simulink model "Xcvr_SSB_AM_2p5"  (Simulink 8.0)
settings: Solver=VariableStepDiscrete  SolverMode=SingleTasking  StartTime=0.0  StopTime=10  RelTol=1e-3
PreLoadFcn:
  | Fs=80e6;
  | 
  | phee=da_rom();
  | [phee_1,phee_2]=da_i2_rom();
  | 
  | Dcic=64;       % CIC decimation
  | Dfac=128;    % following DA filter decimation
  | N = 6;           %       (2^(N+1))=Dfac
  | Daudio=Dcic*Dfac;
  | Faudio=Fs/Daudio;
  | 
  | load info_filt_ssb_4
  | load Serial_Intfc_Stream_5
  | 
  | % AGC related
  | x=0.5:1/256:(1-1/256);
  | addr=(x-0.5)*256;
  | y=1./x;
values from neighbouring files (symbols this model uses):
  Serial_Interface = [0 0 0 0 0 0 0 0 0 0 0 0 ... (11390 elements, 2x5695)]    [Serial_Intfc_Stream_5.mat]
undefined symbols (not defined in the file or in its folder): get, sided, Two, xlipgetpartsetting
undefined symbols (not defined in the file): ssb_coef
libraries: xbsIndex_r4 x1307, dspsrcs4 x5, simulink x2, dspsigops x2, dspsnks4 x1
(part 1 of 11)
settings Model: Creator=dbenson  LastModifiedBy=user
settings DataIOCC: SignalLoggingSaveFormat=ModelDataLogs
settings OptimizationCC: InitFltsAndDblsToZero=on
settings DebuggingCC: FcnCallInpInsideContextMsg=UseLocalSettings  StrictBusMsg=ErrorOnBusTreatedAsVector
settings GRTTargetCC: CombineOutputUpdateFcns=off  GRTInterface=on

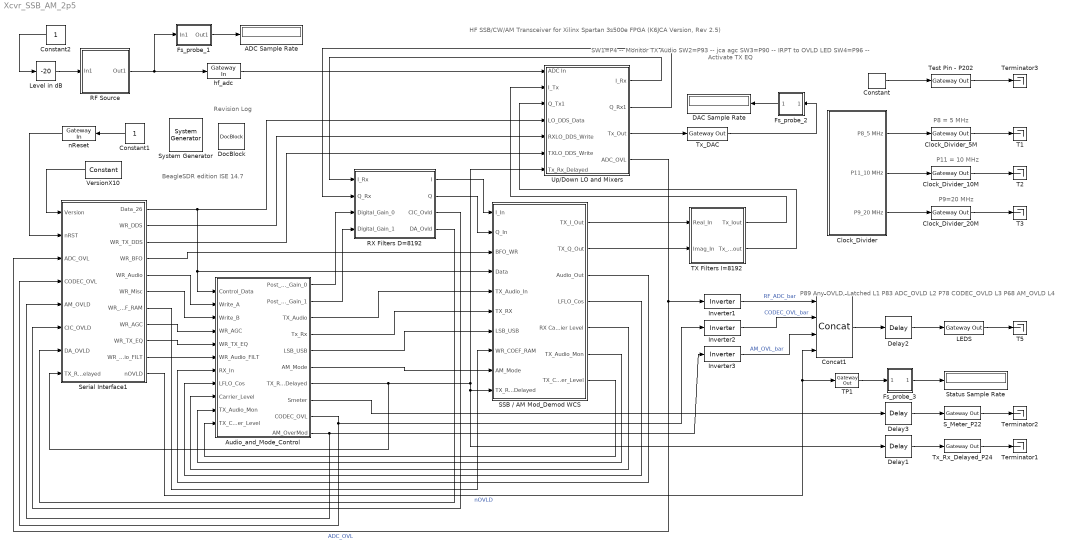
== system Xcvr_SSB_AM_2p5 ==
  note: HF SSB/CW/AM Transceiver for Xilinx Spartan 3s500e FPGA
      | (K6JCA Version, Rev 2.5)
  note: BeagleSDR edition ISE 14.7
  note: SW1=P4 -- Monitor TX Audio
      | SW2=P93 -- jca agc
      | SW3=P90 -- IRPT to OVLD LED
      | SW4=P96 -- Activate TX EQ
  note: P8 = 5 MHz
  note: P11 = 10 MHz
  note: P9=20 MHz
  note: P89  Any OVLD, Latched L1
      | P83  ADC_OVLD L2
      | P78  CODEC_OVLD L3
      | P68  AM_OVLD  L4
  note: Revision
      | Log
  " System Generator" : xbsIndex_r4/ System Generator  Tag=genX  xilinxfamily=spartan3e  part=xc3s500e  speed=-4  package=pq208  synthesis_tool=XST  clock_wrapper=Expose Clock Ports  directory=./netlist_2p5  proj_type=Project Navigator  Synth_file=XST Defaults  Impl_file=ISE Defaults  testbench=off  simulink_period=1/(32*Fs)  sysclk_period=20  dcm_input_clock_period=100  incr_netlist=off  trim_vbits=Everywhere in SubSystem  dbl_ovrd=According to Block Masks  core_generation=According to Block Masks  run_coregen=off  deprecated_control=off  eval_field=0  block_type=sysgen
      settings: block_version=9.2.00
  ADC Sample Rate : Display
  Audio_and_Mode_Control : Subsystem
  Clock_Divider : Subsystem
  Clock_Divider_10M : xbsIndex_r4/Gateway Out  inherit_from_input=off  hdl_port=on  timing_constraint=None  locs_specified=on  LOCs={'P11'}  UseAsDAC=off  DACChannel='1'  block_type=gatewayout
      settings: infoedit="Gateway out block.  Converts Xilinx fixed point inputs into ouputs of type Simulink integer, double, or fixed point.<br><br>Hardware notes:  In hardware these blocks become top level output ports or are discarded, depending on how they are configured."  block_version=12.1
  Clock_Divider_20M : xbsIndex_r4/Gateway Out  inherit_from_input=off  hdl_port=on  timing_constraint=None  locs_specified=on  LOCs={'P9'}  UseAsDAC=off  DACChannel='1'  block_type=gatewayout
      settings: infoedit="Gateway out block.  Converts Xilinx fixed point inputs into ouputs of type Simulink integer, double, or fixed point.<br><br>Hardware notes:  In hardware these blocks become top level output ports or are discarded, depending on how they are configured."  block_version=12.1
  Clock_Divider_5M : xbsIndex_r4/Gateway Out  inherit_from_input=off  hdl_port=on  timing_constraint=None  locs_specified=on  LOCs={'P8'}  UseAsDAC=off  DACChannel='1'  block_type=gatewayout
      settings: infoedit="Gateway out block.  Converts Xilinx fixed point inputs into ouputs of type Simulink integer, double, or fixed point.<br><br>Hardware notes:  In hardware these blocks become top level output ports or are discarded, depending on how they are configured."  block_version=12.1
  Concat1 : xbsIndex_r4/Concat  num_inputs=4  dbl_ovrd=off  block_type=concat
      settings: block_version=12.1
  Constant : xbsIndex_r4/Constant  const=0  gui_display_data_type=Fixed-point  arith_type=Boolean  n_bits=1  bin_pt=0  preci_type=Single  exp_width=8  frac_width=24  explicit_period=off  period=1  equ=P=C  opselect=C  inp2=PCIN>>17  opr=+  inp1=P  carry=CIN  dbl_ovrd=off  block_type=constant
      settings: block_version=12.1
  Constant1 : Constant
  Constant2 : Constant
  DAC Sample Rate : Display
  Delay1 : xbsIndex_r4/Delay  rst=off  infoeditControl=Selection of Reset will increase slice count due to use of real FFs and instead of SRLs  en=off  latency=1  dbl_ovrd=off  reg_retiming=off  block_type=delay
      settings: block_version=12.1
  Delay2 : xbsIndex_r4/Delay  rst=off  infoeditControl=Selection of Reset will increase slice count due to use of real FFs and instead of SRLs  en=off  latency=1  dbl_ovrd=off  reg_retiming=off  block_type=delay
      settings: block_version=12.1
  Delay3 : xbsIndex_r4/Delay  rst=off  infoeditControl=Selection of Reset will increase slice count due to use of real FFs and instead of SRLs  en=off  latency=1  dbl_ovrd=off  reg_retiming=off  block_type=delay
      settings: block_version=12.1
  DocBlock : simulink/Model-Wide Utilities/DocBlock  DocumentType=Text
  Fs_probe_1 : Subsystem
  Fs_probe_2 : Subsystem
  Fs_probe_3 : Subsystem
  Inverter1 : xbsIndex_r4/Inverter  en=off  latency=0  dbl_ovrd=off  block_type=inv
      settings: block_version=12.1
  Inverter2 : xbsIndex_r4/Inverter  en=off  latency=0  dbl_ovrd=off  block_type=inv
      settings: block_version=12.1
  Inverter3 : xbsIndex_r4/Inverter  en=off  latency=0  dbl_ovrd=off  block_type=inv
      settings: block_version=12.1
  LEDS : xbsIndex_r4/Gateway Out  inherit_from_input=off  hdl_port=on  timing_constraint=None  locs_specified=on  LOCs={'P89','P83','P78','P68'}  UseAsDAC=off  DACChannel='1'  block_type=gatewayout
      settings: infoedit="Gateway out block.  Converts Xilinx fixed point inputs into ouputs of type Simulink integer, double, or fixed point.<br><br>Hardware notes:  In hardware these blocks become top level output ports or are discarded, depending on how they are configured."  block_version=12.1
  Level in dB : simulink/Math Operations/Slider Gain  low=-100  gain=-20  high=0
  RF Source : Subsystem
  RX Filters D=8192 : Subsystem
  SSB / AM Mod_Demod WCS : Subsystem
  S_Meter_P22 : xbsIndex_r4/Gateway Out  inherit_from_input=off  hdl_port=on  timing_constraint=None  locs_specified=on  LOCs={'P22'}  UseAsDAC=off  DACChannel='1'  block_type=gatewayout
      settings: infoedit="Gateway out block.  Converts Xilinx fixed point inputs into ouputs of type Simulink integer, double, or fixed point.<br><br>Hardware notes:  In hardware these blocks become top level output ports or are discarded, depending on how they are configured."  block_version=9.2.00
  Serial Interface1 : Subsystem
  Status Sample Rate : Display
  T{1..3,5} (4 alike) : Terminator
  TP1 : xbsIndex_r4/Gateway Out  inherit_from_input=off  hdl_port=off  timing_constraint=None  locs_specified=off  LOCs={ 'b15','c15','c16','d14','b4','e13','k1','g1'}  UseAsDAC=off  DACChannel='1'  block_type=gatewayout
      settings: infoedit="Gateway out block.  Converts Xilinx fixed point inputs into ouputs of type Simulink integer, double, or fixed point.<br><br>Hardware notes:  In hardware these blocks become top level output ports or are discarded, depending on how they are configured."  block_version=9.2.00
  TX Filters I=8192 : Subsystem
  Terminator1 : Terminator
  Terminator2 : Terminator
  Terminator3 : Terminator
  Test Pin - P202 : xbsIndex_r4/Gateway Out  inherit_from_input=off  hdl_port=on  timing_constraint=None  locs_specified=on  LOCs={ 'P202'}  UseAsDAC=off  DACChannel='1'  block_type=gatewayout
      settings: infoedit="Gateway out block.  Converts Xilinx fixed point inputs into ouputs of type Simulink integer, double, or fixed point.<br><br>Hardware notes:  In hardware these blocks become top level output ports or are discarded, depending on how they are configured."  block_version=9.2.00
  Tx_DAC : xbsIndex_r4/Gateway Out  inherit_from_input=off  hdl_port=on  timing_constraint=None  locs_specified=on  LOCs={'P55','P50','P61','P60','P63','P62','P65','P64','P74','P69','P76','P75','P82','P77'}  UseAsDAC=off  DACChannel='1'  block_type=gatewayout
      settings: infoedit="Gateway out block.  Converts Xilinx fixed point inputs into ouputs of type Simulink integer, double, or fixed point.<br><br>Hardware notes:  In hardware these blocks become top level output ports or are discarded, depending on how they are configured."  block_version=12.1
  Tx_Rx_Delayed_P24 : xbsIndex_r4/Gateway Out  inherit_from_input=off  hdl_port=on  timing_constraint=None  locs_specified=on  LOCs={'P24'}  UseAsDAC=off  DACChannel='1'  block_type=gatewayout
      settings: infoedit="Gateway out block.  Converts Xilinx fixed point inputs into ouputs of type Simulink integer, double, or fixed point.<br><br>Hardware notes:  In hardware these blocks become top level output ports or are discarded, depending on how they are configured."  block_version=9.2.00
  Up/Down LO and Mixers : Subsystem
  VersionX10 : xbsIndex_r4/Constant  const=10*2.5  gui_display_data_type=Fixed-point  arith_type=Unsigned  n_bits=8  bin_pt=0  preci_type=Single  exp_width=8  frac_width=24  explicit_period=on  period=8/Fs  equ=P=C  opselect=C  inp2=PCIN>>17  opr=+  inp1=P  carry=CIN  dbl_ovrd=off  block_type=constant
      settings: block_version=12.1
  hf_adc : xbsIndex_r4/Gateway In  gui_display_data_type=Fixed-point  arith_type="Signed  (2's comp)"  n_bits=16  bin_pt=15  preci_type=Single  exp_width=8  frac_width=24  quantization="Round  (unbiased: +/- Inf)"  overflow=Saturate  period=1/Fs  dbl_ovrd=off  timing_constraint=None  locs_specified=on  LOCs="{ 'P186' ,'P185','P181','P180','P179','P178','P177','P172','P171','P168','P167','P165','P164','P163', 'P162',  'P161' }"  UseAsADC=off  ADCChannel='1'  inherit_from_input=off  hdl_port=on  block_type=gatewayin
      settings: infoedit="Gateway in block.  Converts inputs of type Simulink integer, double and fixed point to  Xilinx fixed point type.<br><br>Hardware notes:  In hardware these blocks become top level input ports."  block_version=9.2.00
  nReset : xbsIndex_r4/Gateway In  gui_display_data_type=Fixed-point  arith_type=Boolean  n_bits=1  bin_pt=0  preci_type=Single  exp_width=8  frac_width=24  quantization="Round  (unbiased: +/- Inf)"  overflow=Saturate  period=8/Fs  dbl_ovrd=off  timing_constraint=None  locs_specified=on  LOCs={ 'P101' }  UseAsADC=off  ADCChannel='1'  inherit_from_input=off  hdl_port=on  block_type=gatewayin
      settings: infoedit="Gateway in block.  Converts inputs of type Simulink integer, double and fixed point to  Xilinx fixed point type.<br><br>Hardware notes:  In hardware these blocks become top level input ports."  block_version=9.2.00
  wires:
  Tx_Rx_Delayed_P24/1 -> Terminator1/1
  Serial Interface1/1(Data_26) -> Audio_and_Mode_Control/1(Control_Data), SSB / AM Mod_Demod WCS/4(Data), Up/Down LO and Mixers/4(LO_DDS_Data)
  RX Filters D=8192/2(Q) -> SSB / AM Mod_Demod WCS/2(Q_In)
  SSB / AM Mod_Demod WCS/1(TX_I_Out) -> TX Filters I=8192/1(Real_In)
  SSB / AM Mod_Demod WCS/2(TX_Q_Out) -> TX Filters I=8192/2(Imag_In)
  RX Filters D=8192/1(I) -> SSB / AM Mod_Demod WCS/1(I_In)
  Audio_and_Mode_Control/5(LSB_USB) -> SSB / AM Mod_Demod WCS/7(LSB_USB)
  SSB / AM Mod_Demod WCS/3(Audio_Out) -> Audio_and_Mode_Control/7(RX_In)
  Serial Interface1/5(WR_Audio) -> Audio_and_Mode_Control/2(Write_A)
  Serial Interface1/4(WR_BFO) -> SSB / AM Mod_Demod WCS/3(BFO_WR)
  SSB / AM Mod_Demod WCS/4(LFLO_Cos) -> Audio_and_Mode_Control/8(LFLO_Cos)
  Serial Interface1/6(WR_Misc) -> Audio_and_Mode_Control/3(Write_B)
  RF Source/1(Out1) -> Fs_probe_1/1(In1), hf_adc/1
  Level in dB/1 -> RF Source/1(In1)
  Constant2/1 -> Level in dB/1
  Audio_and_Mode_Control/7(TX_RX_Delayed) -> Up/Down LO and Mixers/7(Tx_Rx_Delayed), SSB / AM Mod_Demod WCS/10(TX_RX_Delayed), Delay1/1, Serial Interface1/8(TX_RX_Delayed)
  Fs_probe_1/1(Out1) -> ADC Sample Rate/1
  Tx_DAC/1 -> Fs_probe_2/1(In1)
  Fs_probe_2/1(Out1) -> DAC Sample Rate/1
  Clock_Divider/1(P8_5 MHz) -> Clock_Divider_5M/1
  Clock_Divider/2(P11_10 MHz) -> Clock_Divider_10M/1
  Clock_Divider/3(P9_20 MHz) -> Clock_Divider_20M/1
  LEDS/1 -> T5/1
  Concat1/1 -> Delay2/1
  hf_adc/1 -> Up/Down LO and Mixers/1(ADC In)
  Audio_and_Mode_Control/6(AM_Mode) -> SSB / AM Mod_Demod WCS/9(AM_Mode)
  Serial Interface1/7(WR_COEF_RAM) -> SSB / AM Mod_Demod WCS/8(WR_COEF_RAM)
  Clock_Divider_5M/1 -> T1/1
  Clock_Divider_10M/1 -> T2/1
  Clock_Divider_20M/1 -> T3/1
  VersionX10/1 -> Serial Interface1/1(Version)
  Fs_probe_3/1(Out1) -> Status Sample Rate/1
  TP1/1 -> Fs_probe_3/1(In1)
  Audio_and_Mode_Control/9(CODEC_OVL) -> Serial Interface1/4(CODEC_OVL), Inverter2/1
  Serial Interface1/11(nOVLD) -> TP1/1, Concat1/4  "nOVLD"
  Serial Interface1/2(WR_DDS) -> Up/Down LO and Mixers/5(RXLO_DDS_Write)
  Up/Down LO and Mixers/3(Tx_Out) -> Tx_DAC/1
  Up/Down LO and Mixers/1(I_Rx) -> RX Filters D=8192/1(I_Rx)
  Up/Down LO and Mixers/2(Q_Rx1) -> RX Filters D=8192/2(Q_Rx)
  TX Filters I=8192/1(Tx_Iout) -> Up/Down LO and Mixers/2(I_Tx)
  TX Filters I=8192/2(Tx_Qout) -> Up/Down LO and Mixers/3(Q_Tx1)
  SSB / AM Mod_Demod WCS/5(RX Carrier Level) -> Audio_and_Mode_Control/9(Carrier_Level)
  Audio_and_Mode_Control/10(AM_OverMod) -> Inverter3/1, Serial Interface1/5(AM_OVLD)
  Inverter1/1 -> Concat1/1  "RF_ADC_bar"
  Inverter2/1 -> Concat1/2  "CODEC_OVL_bar"
  Inverter3/1 -> Concat1/3  "AM_OVL_bar"
  Delay1/1 -> Tx_Rx_Delayed_P24/1
  Delay2/1 -> LEDS/1
  RX Filters D=8192/3(CIC_Ovld) -> Serial Interface1/6(CIC_OVLD)
  RX Filters D=8192/4(DA_Ovld) -> Serial Interface1/7(DA_OVLD)
  Audio_and_Mode_Control/8(Smeter) -> Delay3/1
  Up/Down LO and Mixers/4(ADC_OVL) -> Inverter1/1, Serial Interface1/3(ADC_OVL)  "ADC_OVL"
  Serial Interface1/8(WR_AGC) -> Audio_and_Mode_Control/4(WR_AGC)
  Audio_and_Mode_Control/3(TX_Audio) -> SSB / AM Mod_Demod WCS/5(TX_Audio_In)
  nReset/1 -> Serial Interface1/2(nRST)
  Serial Interface1/3(WR_TX_DDS) -> Up/Down LO and Mixers/6(TXLO_DDS_Write)
  SSB / AM Mod_Demod WCS/7(TX_Carrier_Level) -> Audio_and_Mode_Control/11(TX_Carrier_Level)
  SSB / AM Mod_Demod WCS/6(TX_Audio_Mon) -> Audio_and_Mode_Control/10(TX_Audio_Mon)
  Constant1/1 -> nReset/1
  Audio_and_Mode_Control/4(Tx_Rx) -> SSB / AM Mod_Demod WCS/6(TX_RX)
  S_Meter_P22/1 -> Terminator2/1
  Delay3/1 -> S_Meter_P22/1
  Test Pin - P202/1 -> Terminator3/1
  Constant/1 -> Test Pin - P202/1
  Serial Interface1/10(WR_Audio_FILT) -> Audio_and_Mode_Control/6(WR_Audio_FILT)
  Serial Interface1/9(WR_TX_EQ) -> Audio_and_Mode_Control/5(WR_TX_EQ)
  Audio_and_Mode_Control/1(Post_CIC_Gain_0) -> RX Filters D=8192/3(Digital_Gain_0)
  Audio_and_Mode_Control/2(Post_CIC_Gain_1) -> RX Filters D=8192/4(Digital_Gain_1)

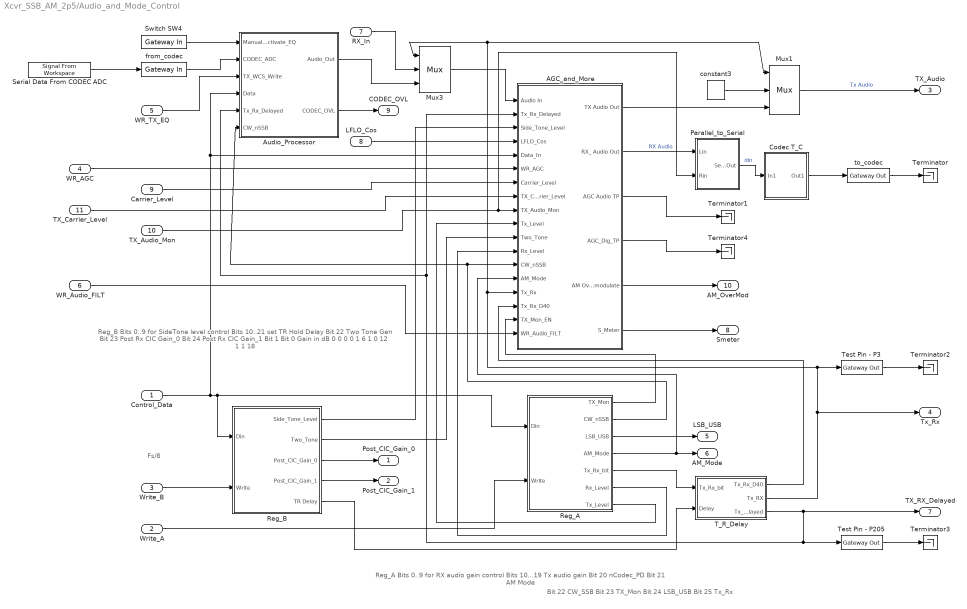
== system Xcvr_SSB_AM_2p5/Audio_and_Mode_Control ==
  note: Fs/8
  note: Reg_A
      | Bits 0..9 for RX audio gain control
      | Bits 10...19 Tx audio gain
      | Bit 20 nCodec_PD
      | Bit 21 AM Mode
  note: Reg_B
      | Bits 0..9 for SideTone level control
      | Bits 10..21 set TR Hold Delay
      | Bit 22 Two Tone Gen
      | Bit 23 Post Rx CIC Gain_0
      | Bit 24 Post Rx CIC Gain_1
      |            Bit 1  Bit 0   Gain in dB
      |               0      0         0
      |               0      1         6
      |               1      0        12
      |               1      1        18
  note: Bit 22 CW_SSB
      | Bit 23 TX_Mon
      | Bit 24 LSB_USB
      | Bit 25 Tx_Rx
  Control_Data : Inport
  Write_A : Inport  Port=2
  Write_B : Inport  Port=3
  WR_AGC : Inport  Port=4
  WR_TX_EQ : Inport  Port=5
  WR_Audio_FILT : Inport  Port=6
  RX_In : Inport  Port=7
  LFLO_Cos : Inport  Port=8
  Carrier_Level : Inport  Port=9
  TX_Audio_Mon : Inport  Port=10
  TX_Carrier_Level : Inport  Port=11
  AGC_and_More : Subsystem
  Audio_Processor : Subsystem
  Codec T_C : Subsystem
  Mux1 : xbsIndex_r4/Mux  inputs=2  en=off  latency=0  precision=Full  arith_type=Unsigned  n_bits=32  bin_pt=32  quantization="Round  (unbiased: +/- Inf)"  overflow=Wrap  dbl_ovrd=off  block_type=mux
      settings: block_version=9.2.00
  Mux3 : xbsIndex_r4/Mux  inputs=2  en=off  latency=0  precision=Full  arith_type=Unsigned  n_bits=32  bin_pt=32  quantization="Round  (unbiased: +/- Inf)"  overflow=Wrap  dbl_ovrd=off  block_type=mux
      settings: block_version=9.2.00
  Parallel_to_Serial : Subsystem
  Reg_A : Subsystem
  Reg_B : Subsystem
  Serial Data From CODEC ADC : dspsrcs4/Signal From Workspace  X=[[ 0 1 1 1 1 0 0 0 0 0 0 0 0 0 0 0 ],[1 1 0 0 0 0 0 0 0 0 0 0 0 0 0 0]]  Ts=256/Fs  nsamps=1  OutputAfterFinalValue=Cyclic repetition  ignoreOrWarnInputAndFrameLengths=off
  Switch SW4 : xbsIndex_r4/Gateway In  gui_display_data_type=Fixed-point  arith_type=Boolean  n_bits=1  bin_pt=0  preci_type=Single  exp_width=8  frac_width=24  quantization="Round  (unbiased: +/- Inf)"  overflow=Saturate  period=1/Faudio  dbl_ovrd=off  timing_constraint=None  locs_specified=on  LOCs={'P96'}  UseAsADC=off  ADCChannel='1'  inherit_from_input=off  hdl_port=on  block_type=gatewayin
      settings: infoedit="Gateway in block.  Converts inputs of type Simulink integer, double and fixed point to  Xilinx fixed point type.<br><br>Hardware notes:  In hardware these blocks become top level input ports."  block_version=9.2.00
  T_R_Delay : Subsystem
  Terminator{,1..4} (5 alike) : Terminator
  Test Pin - P205 : xbsIndex_r4/Gateway Out  inherit_from_input=off  hdl_port=on  timing_constraint=None  locs_specified=on  LOCs={ 'P205'}  UseAsDAC=off  DACChannel='1'  block_type=gatewayout
      settings: infoedit="Gateway out block.  Converts Xilinx fixed point inputs into ouputs of type Simulink integer, double, or fixed point.<br><br>Hardware notes:  In hardware these blocks become top level output ports or are discarded, depending on how they are configured."  block_version=9.2.00
  Test Pin - P3 : xbsIndex_r4/Gateway Out  inherit_from_input=off  hdl_port=on  timing_constraint=None  locs_specified=on  LOCs={ 'P3'}  UseAsDAC=off  DACChannel='1'  block_type=gatewayout
      settings: infoedit="Gateway out block.  Converts Xilinx fixed point inputs into ouputs of type Simulink integer, double, or fixed point.<br><br>Hardware notes:  In hardware these blocks become top level output ports or are discarded, depending on how they are configured."  block_version=9.2.00
  constant3 : xbsIndex_r4/Constant  const=0  gui_display_data_type=Fixed-point  arith_type=Signed (2's comp)  n_bits=16  bin_pt=15  preci_type=Single  exp_width=8  frac_width=24  explicit_period=on  period=8192/Fs  equ=P=C  opselect=C  inp2=PCIN>>17  opr=+  inp1=P  carry=CIN  dbl_ovrd=off  block_type=constant
      settings: block_version=9.2.00
  from_codec : xbsIndex_r4/Gateway In  gui_display_data_type=Fixed-point  arith_type=Unsigned  n_bits=1  bin_pt=0  preci_type=Single  exp_width=8  frac_width=24  quantization="Round  (unbiased: +/- Inf)"  overflow=Saturate  period=256/Fs  dbl_ovrd=off  timing_constraint=None  locs_specified=on  LOCs={'P146'}  UseAsADC=off  ADCChannel='1'  inherit_from_input=off  hdl_port=on  block_type=gatewayin
      settings: infoedit="Gateway in block.  Converts inputs of type Simulink integer, double and fixed point to  Xilinx fixed point type.<br><br>Hardware notes:  In hardware these blocks become top level input ports."  block_version=9.2.00
  to_codec : xbsIndex_r4/Gateway Out  inherit_from_input=off  hdl_port=on  timing_constraint=None  locs_specified=on  LOCs={ 'P153', 'P152','P151','P150','P147'}  UseAsDAC=off  DACChannel='1'  block_type=gatewayout
      settings: infoedit="Gateway out block.  Converts Xilinx fixed point inputs into ouputs of type Simulink integer, double, or fixed point.<br><br>Hardware notes:  In hardware these blocks become top level output ports or are discarded, depending on how they are configured."  block_version=9.2.00
  Post_CIC_Gain_0 : Outport
  Post_CIC_Gain_1 : Outport  Port=2
  TX_Audio : Outport  Port=3
  Tx_Rx : Outport  Port=4
  LSB_USB : Outport  Port=5
  AM_Mode : Outport  Port=6
  TX_RX_Delayed : Outport  Port=7
  Smeter : Outport  Port=8
  CODEC_OVL : Outport  Port=9
  AM_OverMod : Outport  Port=10
  wires:
  Reg_A/3(LSB_USB) -> LSB_USB/1
  Codec T_C/1(Out1) -> to_codec/1
  to_codec/1 -> Terminator/1
  Serial Data From CODEC ADC/1 -> from_codec/1
  Write_A/1 -> Reg_A/2(Write)
  Control_Data/1 -> Reg_B/1(Din), Reg_A/1(Din), Audio_Processor/4(Data), AGC_and_More/5(Data_In)
  constant3/1 -> Mux1/2
  RX_In/1 -> Mux3/2
  Mux3/1 -> AGC_and_More/1(Audio In)
  Mux1/1 -> TX_Audio/1  "Tx Audio"
  Write_B/1 -> Reg_B/2(Write)
  AGC_and_More/1(TX Audio Out) -> Mux1/3
  Reg_B/1(Side_Tone_Level) -> AGC_and_More/3(Side_Tone_Level)
  T_R_Delay/3(Tx_RX_Delayed) -> TX_RX_Delayed/1, AGC_and_More/2(Tx_Rx_Delayed), Audio_Processor/5(Tx_Rx_Delayed), Test Pin - P205/1
  Reg_B/5(TR Delay) -> T_R_Delay/2(Delay)
  Reg_B/2(Two_Tone) -> AGC_and_More/11(Two_Tone)
  Reg_A/7(Tx_Level) -> AGC_and_More/10(Tx_Level)
  Reg_A/6(Rx_Level) -> AGC_and_More/12(Rx_Level)
  Reg_A/4(AM_Mode) -> AGC_and_More/14(AM_Mode), AM_Mode/1
  Reg_B/3(Post_CIC_Gain_0) -> Post_CIC_Gain_0/1
  Reg_B/4(Post_CIC_Gain_1) -> Post_CIC_Gain_1/1
  AGC_and_More/3(AGC Audio TP) -> Terminator1/1
  WR_AGC/1 -> AGC_and_More/6(WR_AGC)
  T_R_Delay/2(Tx_RX) -> Tx_Rx/1, Mux3/1, Mux1/1, AGC_and_More/15(Tx_Rx), Test Pin - P3/1
  Reg_A/5(Tx_Rx_bit) -> T_R_Delay/1(Tx_Rx_bit)
  Parallel_to_Serial/1(Serial_Out) -> Codec T_C/1(In1)  "din"
  Audio_Processor/1(Audio_Out) -> Mux3/3
  from_codec/1 -> Audio_Processor/2(CODEC_ADC)
  Audio_Processor/2(CODEC_OVL) -> CODEC_OVL/1
  Switch SW4/1 -> Audio_Processor/1(Manual_Activate_EQ)
  AGC_and_More/4(AGC_Dig_TP) -> Terminator4/1
  TX_Carrier_Level/1 -> AGC_and_More/8(TX_Carrier_Level)
  AGC_and_More/5(AM Overmodulate) -> AM_OverMod/1
  AGC_and_More/2(RX_ Audio Out) -> Parallel_to_Serial/1(Lin)  "RX Audio"
  TX_Audio_Mon/1 -> AGC_and_More/9(TX_Audio_Mon), Parallel_to_Serial/2(Rin)
  T_R_Delay/1(Tx_Rx_D40) -> AGC_and_More/16(Tx_Rx_D40)
  Reg_A/2(CW_nSSB) -> AGC_and_More/13(CW_nSSB), Audio_Processor/6(CW_nSSB)
  WR_TX_EQ/1 -> Audio_Processor/3(TX_WCS_Write)
  AGC_and_More/6(S_Meter) -> Smeter/1
  Reg_A/1(TX_Mon) -> AGC_and_More/17(TX_Mon_EN)
  Test Pin - P3/1 -> Terminator2/1
  Test Pin - P205/1 -> Terminator3/1
  Carrier_Level/1 -> AGC_and_More/7(Carrier_Level)
  LFLO_Cos/1 -> AGC_and_More/4(LFLO_Cos)
  WR_Audio_FILT/1 -> AGC_and_More/18(WR_Audio_FILT)

== system Xcvr_SSB_AM_2p5/Clock_Divider ==
  Counter : xbsIndex_r4/Counter  cnt_type=Free Running  cnt_to=Inf  operation=Up  start_count=0  cnt_by_val=1  arith_type=Unsigned  n_bits=4  bin_pt=0  load_pin=off  rst=off  en=off  explicit_period=on  period=1/Fs  dbl_ovrd=off  use_behavioral_HDL=off  implementation=Fabric  block_type=counter
      settings: block_version=12.1
  Register3 : xbsIndex_r4/Register  init=0  rst=off  en=off  dbl_ovrd=off  block_type=register
      settings: block_version=12.1
  Register4 : xbsIndex_r4/Register  init=0  rst=off  en=off  dbl_ovrd=off  block_type=register
      settings: block_version=12.1
  Register5 : xbsIndex_r4/Register  init=0  rst=off  en=off  dbl_ovrd=off  block_type=register
      settings: block_version=12.1
  Slice - bit 2 : xbsIndex_r4/Slice  nbits=1  boolean_output=off  mode=Upper Bit Location + Width  bit1=-2  base1=MSB of Input  bit0=0  base0=LSB of Input  dbl_ovrd=off  block_type=slice
      settings: block_version=12.1
  Slice - bit 3 : xbsIndex_r4/Slice  nbits=1  boolean_output=off  mode=Upper Bit Location + Width  bit1=-1  base1=MSB of Input  bit0=0  base0=LSB of Input  dbl_ovrd=off  block_type=slice
      settings: block_version=12.1
  Slice - bit 4 : xbsIndex_r4/Slice  nbits=1  boolean_output=off  mode=Upper Bit Location + Width  bit1=0  base1=MSB of Input  bit0=0  base0=LSB of Input  dbl_ovrd=off  block_type=slice
      settings: block_version=12.1
  P8_5 MHz : Outport
  P11_10 MHz : Outport  Port=2
  P9_20 MHz : Outport  Port=3
  wires:
  Register3/1 -> P8_5 MHz/1  "5_MHz"
  Counter/1 -> Slice - bit 4/1, Slice - bit 3/1, Slice - bit 2/1
  Slice - bit 4/1 -> Register3/1  "5MHz"
  Slice - bit 3/1 -> Register5/1  "10 MHz"
  Slice - bit 2/1 -> Register4/1  "20 MHz"
  Register4/1 -> P9_20 MHz/1  "20_MHz"
  Register5/1 -> P11_10 MHz/1

== system Xcvr_SSB_AM_2p5/Fs_probe_1 ==
  In1 : Inport
  Probe : Probe  ProbeWidth=off  ProbeComplexSignal=off
  Product : Product  Inputs=/  RndMeth=Zero
  Selector : Selector  InputPortWidth=2  IndexOptions=Index vector (dialog)  Indices=1  OutputSizes=1
  Out1 : Outport
  wires:
  Selector/1 -> Product/1
  Probe/1 -> Selector/1
  In1/1 -> Probe/1
  Product/1 -> Out1/1

== system Xcvr_SSB_AM_2p5/Fs_probe_2 ==
  In1 : Inport
  Probe : Probe  ProbeWidth=off  ProbeComplexSignal=off
  Product : Product  Inputs=/  RndMeth=Zero
  Selector : Selector  InputPortWidth=2  IndexOptions=Index vector (dialog)  Indices=1  OutputSizes=1
  Out1 : Outport
  wires:
  Product/1 -> Out1/1
  In1/1 -> Probe/1
  Probe/1 -> Selector/1
  Selector/1 -> Product/1

== system Xcvr_SSB_AM_2p5/Fs_probe_3 ==
  In1 : Inport
  Probe : Probe  ProbeWidth=off  ProbeComplexSignal=off
  Product : Product  Inputs=/  RndMeth=Zero
  Selector : Selector  InputPortWidth=2  IndexOptions=Index vector (dialog)  Indices=1  OutputSizes=1
  Out1 : Outport
  wires:
  Product/1 -> Out1/1
  In1/1 -> Probe/1
  Probe/1 -> Selector/1
  Selector/1 -> Product/1

== system Xcvr_SSB_AM_2p5/RF Source ==
  In1 : Inport
  ADC DC Offset : Constant  Value=0
  Add : Sum  Inputs=+++
  Gain : Gain  Gain=1/20
  Math Function : Math  Operator=10^u  SaturateOnIntegerOverflow=on
  Product1 : Product  RndMeth=Zero
  Random Source : dspsrcs4/Random Source  SrcType=Gaussian  NormMethod=Ziggurat  CltLength=12  MinVal=0  MaxVal=1  MeanVal=0  VarVal=0.0001*.0005^2  RepMode=Not repeatable  rawSeed=1  IsInherit=off  SampMode=Discrete  SampTime=1/Fs  SampFrame=1  DataType=Double  OutComplex=Real
  Sine Wave : dspsrcs4/Sine Wave  Amplitude=.99  Frequency=10.001e6  Phase=0  SampleMode=Discrete  OutComplex=Real  CompMethod=Trigonometric fcn  TableSize=Speed  SampleTime=1/Fs  SamplesPerFrame=1  ResetState=Restart at time zero  dataType=double  wordLen=16  udDataType=sfix(16)  fracBitsMode=Best precision  numFracBits=15  OutDataTypeStr=double  LastOutDataTypeStr=double
  Out1 : Outport
  wires:
  In1/1 -> Gain/1
  Math Function/1 -> Product1/2
  Gain/1 -> Math Function/1
  Sine Wave/1 -> Product1/1
  Product1/1 -> Add/1
  Add/1 -> Out1/1
  ADC DC Offset/1 -> Add/2
  Random Source/1 -> Add/3

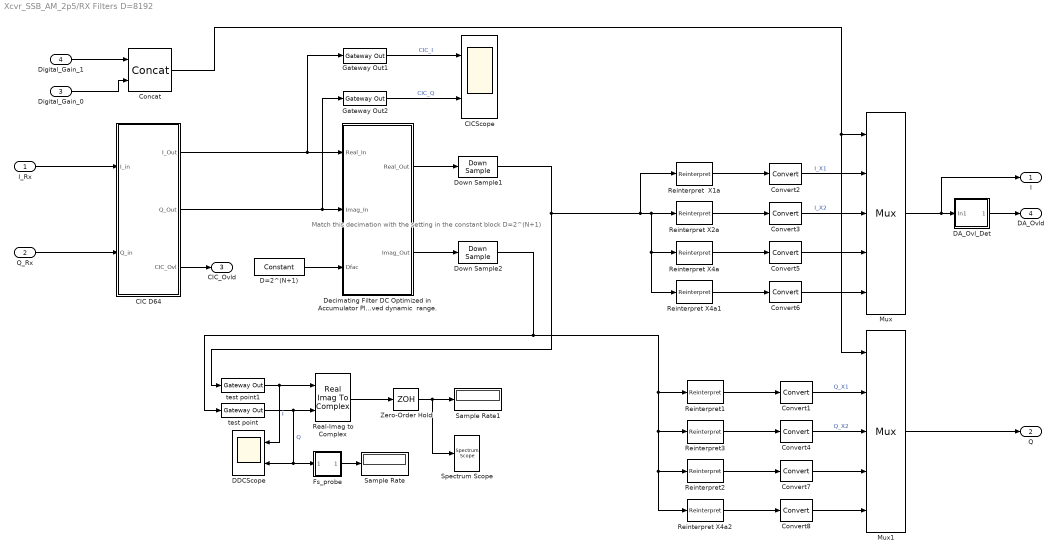
== system Xcvr_SSB_AM_2p5/RX Filters D=8192 ==
  note: Match this decimation
      |  with the setting in the
      | constant block D=2^(N+1)
  I_Rx : Inport
  Q_Rx : Inport  Port=2
  Digital_Gain_0 : Inport  Port=3
  Digital_Gain_1 : Inport  Port=4
  CIC D64 : Subsystem
  CICScope : Scope  NumInputPorts=2
      settings: TimeRange=5e-006  YMin=-0.75~-1  YMax=0.75~1  MaxDataPoints=50000
  Concat : xbsIndex_r4/Concat  num_inputs=2  dbl_ovrd=off  block_type=concat
      settings: block_version=12.1
  Convert{1..8} (8 alike) : xbsIndex_r4/Convert  gui_display_data_type=Fixed-point  arith_type="Signed  (2's comp)"  n_bits=18  bin_pt=17  float_type=Single  exp_bits=8  fraction_bits=24  quantization="Round  (unbiased: +/- Inf)"  overflow=Saturate  en=off  latency=1  dbl_ovrd=off  pipeline=off  block_type=convert
      settings: block_version=9.2.00
  D=2^(N+1) : xbsIndex_r4/Constant  const=N  gui_display_data_type=Fixed-point  arith_type=Unsigned  n_bits=3  bin_pt=0  preci_type=Single  exp_width=8  frac_width=24  explicit_period=off  period=1  equ=P=C  opselect=C  inp2=PCIN>>17  opr=+  inp1=P  carry=CIN  dbl_ovrd=off  block_type=constant
      settings: block_version=9.2.00
  DA_Ovl_Det : Subsystem
  DDCScope : Scope  NumInputPorts=2
      settings: TimeRange=0.02  YMin=-1~-0.75  YMax=1~0.75  SaveName=ScopeData2  MaxDataPoints=50000
  "Decimating Filter DC Optimized in Accumulator Plus Pipelined Stage Control. Improved dynamic  range. " : Subsystem
  Down Sample1 : xbsIndex_r4/Down Sample  sample_ratio=128  sample_phase="Last Value of Frame  (most efficient)"  en=off  latency=1  dbl_ovrd=off  block_type=dsamp
      settings: block_version=9.2.00
  Down Sample2 : xbsIndex_r4/Down Sample  sample_ratio=128  sample_phase="Last Value of Frame  (most efficient)"  en=off  latency=1  dbl_ovrd=off  block_type=dsamp
      settings: block_version=9.2.00
  Fs_probe : Subsystem
  Gateway Out1 : xbsIndex_r4/Gateway Out  inherit_from_input=off  hdl_port=off  timing_constraint=None  locs_specified=off  LOCs={}  UseAsDAC=off  DACChannel='1'  block_type=gatewayout
      settings: infoedit="Gateway out block.  Converts Xilinx fixed point inputs into ouputs of type Simulink integer, double, or fixed point.<P><P>Hardware notes:  In hardware these blocks become top level output ports or are discarded, depending on how they are configured."  block_version=9.2.00
  Gateway Out2 : xbsIndex_r4/Gateway Out  inherit_from_input=off  hdl_port=off  timing_constraint=None  locs_specified=off  LOCs={}  UseAsDAC=off  DACChannel='1'  block_type=gatewayout
      settings: infoedit="Gateway out block.  Converts Xilinx fixed point inputs into ouputs of type Simulink integer, double, or fixed point.<P><P>Hardware notes:  In hardware these blocks become top level output ports or are discarded, depending on how they are configured."  block_version=9.2.00
  Mux : xbsIndex_r4/Mux  inputs=4  en=off  latency=0  precision=Full  arith_type=Unsigned  n_bits=16  bin_pt=14  quantization=Truncate  overflow=Wrap  dbl_ovrd=off  block_type=mux
      settings: block_version=12.1
  Mux1 : xbsIndex_r4/Mux  inputs=4  en=off  latency=0  precision=Full  arith_type=Unsigned  n_bits=16  bin_pt=14  quantization=Truncate  overflow=Wrap  dbl_ovrd=off  block_type=mux
      settings: block_version=12.1
  Real-Imag to Complex : RealImagToComplex
  Reinterpret  X1a : xbsIndex_r4/Reinterpret  force_arith_type=on  arith_type="Signed  (2's comp)"  force_bin_pt=on  bin_pt=20  block_type=reinterpret
      settings: infoedit="Changes signal type without altering the binary representation.   You can changed the signal between signed and unsigned, and relocate the binary point.<br><br>Hardware notes: In hardware this block costs nothing.<br><br>Example:  Suppose the input is 6 bits wide, signed, with 2 fractional bits, and the output is forced to unsigned with 0 fractional bits.  Then an input of -2.0 (1110.00 in binary 2's complement) becomes an output of 56 (111000 in binary)."  block_version=9.2.00
  Reinterpret X2a : xbsIndex_r4/Reinterpret  force_arith_type=on  arith_type="Signed  (2's comp)"  force_bin_pt=on  bin_pt=19  block_type=reinterpret
      settings: infoedit="Changes signal type without altering the binary representation.   You can changed the signal between signed and unsigned, and relocate the binary point.<br><br>Hardware notes: In hardware this block costs nothing.<br><br>Example:  Suppose the input is 6 bits wide, signed, with 2 fractional bits, and the output is forced to unsigned with 0 fractional bits.  Then an input of -2.0 (1110.00 in binary 2's complement) becomes an output of 56 (111000 in binary)."  block_version=9.2.00
  Reinterpret X4a : xbsIndex_r4/Reinterpret  force_arith_type=on  arith_type="Signed  (2's comp)"  force_bin_pt=on  bin_pt=18  block_type=reinterpret
      settings: infoedit="Changes signal type without altering the binary representation.   You can changed the signal between signed and unsigned, and relocate the binary point.<br><br>Hardware notes: In hardware this block costs nothing.<br><br>Example:  Suppose the input is 6 bits wide, signed, with 2 fractional bits, and the output is forced to unsigned with 0 fractional bits.  Then an input of -2.0 (1110.00 in binary 2's complement) becomes an output of 56 (111000 in binary)."  block_version=9.2.00
  Reinterpret X4a1 : xbsIndex_r4/Reinterpret  force_arith_type=on  arith_type="Signed  (2's comp)"  force_bin_pt=on  bin_pt=17  block_type=reinterpret
      settings: infoedit="Changes signal type without altering the binary representation.   You can changed the signal between signed and unsigned, and relocate the binary point.<br><br>Hardware notes: In hardware this block costs nothing.<br><br>Example:  Suppose the input is 6 bits wide, signed, with 2 fractional bits, and the output is forced to unsigned with 0 fractional bits.  Then an input of -2.0 (1110.00 in binary 2's complement) becomes an output of 56 (111000 in binary)."  block_version=9.2.00
  Reinterpret X4a2 : xbsIndex_r4/Reinterpret  force_arith_type=on  arith_type="Signed  (2's comp)"  force_bin_pt=on  bin_pt=17  block_type=reinterpret
      settings: infoedit="Changes signal type without altering the binary representation.   You can changed the signal between signed and unsigned, and relocate the binary point.<br><br>Hardware notes: In hardware this block costs nothing.<br><br>Example:  Suppose the input is 6 bits wide, signed, with 2 fractional bits, and the output is forced to unsigned with 0 fractional bits.  Then an input of -2.0 (1110.00 in binary 2's complement) becomes an output of 56 (111000 in binary)."  block_version=9.2.00
  Reinterpret1 : xbsIndex_r4/Reinterpret  force_arith_type=on  arith_type="Signed  (2's comp)"  force_bin_pt=on  bin_pt=20  block_type=reinterpret
      settings: infoedit="Changes signal type without altering the binary representation.   You can changed the signal between signed and unsigned, and relocate the binary point.<br><br>Hardware notes: In hardware this block costs nothing.<br><br>Example:  Suppose the input is 6 bits wide, signed, with 2 fractional bits, and the output is forced to unsigned with 0 fractional bits.  Then an input of -2.0 (1110.00 in binary 2's complement) becomes an output of 56 (111000 in binary)."  block_version=9.2.00
  Reinterpret2 : xbsIndex_r4/Reinterpret  force_arith_type=on  arith_type="Signed  (2's comp)"  force_bin_pt=on  bin_pt=18  block_type=reinterpret
      settings: infoedit="Changes signal type without altering the binary representation.   You can changed the signal between signed and unsigned, and relocate the binary point.<br><br>Hardware notes: In hardware this block costs nothing.<br><br>Example:  Suppose the input is 6 bits wide, signed, with 2 fractional bits, and the output is forced to unsigned with 0 fractional bits.  Then an input of -2.0 (1110.00 in binary 2's complement) becomes an output of 56 (111000 in binary)."  block_version=9.2.00
  Reinterpret3 : xbsIndex_r4/Reinterpret  force_arith_type=on  arith_type="Signed  (2's comp)"  force_bin_pt=on  bin_pt=19  block_type=reinterpret
      settings: infoedit="Changes signal type without altering the binary representation.   You can changed the signal between signed and unsigned, and relocate the binary point.<br><br>Hardware notes: In hardware this block costs nothing.<br><br>Example:  Suppose the input is 6 bits wide, signed, with 2 fractional bits, and the output is forced to unsigned with 0 fractional bits.  Then an input of -2.0 (1110.00 in binary 2's complement) becomes an output of 56 (111000 in binary)."  block_version=9.2.00
  Sample Rate : Display
  Sample Rate1 : Display
  Spectrum Scope : dspsnks4/Spectrum Scope  ScopeProperties=on  Domain=Frequency  HorizSpan=1  UseBuffer=off  BufferSize=128  Overlap=0  TreatMby1Signals=One channel  inpFftLenInherit=off  FFTlength=128  numAvg=2  DisplayProperties=off  AxisGrid=on  Memory=off  FrameNumber=on  AxisLegend=off  AxisZoom=off  OpenScopeAtSimStart=on  OpenScopeImmediately=off  FigPos=get(0,'defaultfigureposition')  AxisProperties=off  XUnits=Hertz  XRange=Two-sided ((-Fs/2...Fs/2])  XDisplay=0  InheritXIncr=on  XIncr=1.0  XLabel=Samples  XLimit=Auto  YUnits=dBW/Hertz  XMax=1  XMin=0  YLabel=Magnitude-squared, dB  LineProperties=off  wintypeSpecScope=Hann  RsSpecScope=50  betaSpecScope=5  winsampSpecScope=Periodic  XAxisParamsVer=6.9  isFrameUpgraded=on
      settings: YMin=-10  YMax=10
  Zero-Order Hold : ZeroOrderHold  SampleTime=Dcic*Dfac/Fs
  test point : xbsIndex_r4/Gateway Out  inherit_from_input=off  hdl_port=off  timing_constraint=None  locs_specified=off  LOCs={'a222'}  UseAsDAC=off  DACChannel='1'  block_type=gatewayout
      settings: infoedit="Gateway out block.  Converts Xilinx fixed point inputs into ouputs of type Simulink integer, double, or fixed point.<P><P>Hardware notes:  In hardware these blocks become top level output ports or are discarded, depending on how they are configured."  block_version=9.2.00
  test point1 : xbsIndex_r4/Gateway Out  inherit_from_input=off  hdl_port=off  timing_constraint=None  locs_specified=off  LOCs={'a222'}  UseAsDAC=off  DACChannel='1'  block_type=gatewayout
      settings: infoedit="Gateway out block.  Converts Xilinx fixed point inputs into ouputs of type Simulink integer, double, or fixed point.<P><P>Hardware notes:  In hardware these blocks become top level output ports or are discarded, depending on how they are configured."  block_version=9.2.00
  I : Outport
  Q : Outport  Port=2
  CIC_Ovld : Outport  Port=3
  DA_Ovld : Outport  Port=4
  wires:
  D=2^(N+1)/1 -> "Decimating Filter DC Optimized in Accumulator Plus Pipelined Stage Control. Improved dynamic  range. "/3(Dfac)
  Gateway Out2/1 -> CICScope/2  "CIC_Q"
  Down Sample1/1 -> test point1/1, Reinterpret X2a/1, Reinterpret X4a/1, Reinterpret X4a1/1, Reinterpret  X1a/1
  Down Sample2/1 -> test point/1, Reinterpret1/1, Reinterpret3/1, Reinterpret2/1, Reinterpret X4a2/1
  test point1/1 -> Real-Imag to Complex/1, DDCScope/1  "I"
  test point/1 -> Real-Imag to Complex/2, DDCScope/2, Fs_probe/1(In1)  "Q"
  Real-Imag to Complex/1 -> Zero-Order Hold/1
  Fs_probe/1(Out1) -> Sample Rate/1
  Zero-Order Hold/1 -> Spectrum Scope/1, Sample Rate1/1
  CIC D64/1(I_Out) -> Gateway Out1/1, "Decimating Filter DC Optimized in Accumulator Plus Pipelined Stage Control. Improved dynamic  range. "/1(Real_In)
  CIC D64/2(Q_Out) -> Gateway Out2/1, "Decimating Filter DC Optimized in Accumulator Plus Pipelined Stage Control. Improved dynamic  range. "/2(Imag_In)
  "Decimating Filter DC Optimized in Accumulator Plus Pipelined Stage Control. Improved dynamic  range. "/1(Real_Out) -> Down Sample1/1
  "Decimating Filter DC Optimized in Accumulator Plus Pipelined Stage Control. Improved dynamic  range. "/2(Imag_Out) -> Down Sample2/1
  Q_Rx/1 -> CIC D64/2(Q_in)
  I_Rx/1 -> CIC D64/1(I_in)
  Gateway Out1/1 -> CICScope/1  "CIC_I"
  DA_Ovl_Det/1(Out1) -> DA_Ovld/1
  CIC D64/3(CIC_Ovl) -> CIC_Ovld/1
  Digital_Gain_0/1 -> Concat/2
  Digital_Gain_1/1 -> Concat/1
  Reinterpret  X1a/1 -> Convert2/1
  Reinterpret X2a/1 -> Convert3/1
  Convert3/1 -> Mux/3  "I_X2"
  Convert2/1 -> Mux/2  "I_X1"
  Reinterpret1/1 -> Convert1/1
  Reinterpret3/1 -> Convert4/1
  Reinterpret X4a/1 -> Convert5/1
  Convert5/1 -> Mux/4
  Convert1/1 -> Mux1/2  "Q_X1"
  Convert4/1 -> Mux1/3  "Q_X2"
  Convert7/1 -> Mux1/4
  Reinterpret2/1 -> Convert7/1
  Mux1/1 -> Q/1
  Mux/1 -> DA_Ovl_Det/1(In1), I/1
  Concat/1 -> Mux/1, Mux1/1
  Reinterpret X4a1/1 -> Convert6/1
  Convert6/1 -> Mux/5
  Reinterpret X4a2/1 -> Convert8/1
  Convert8/1 -> Mux1/5

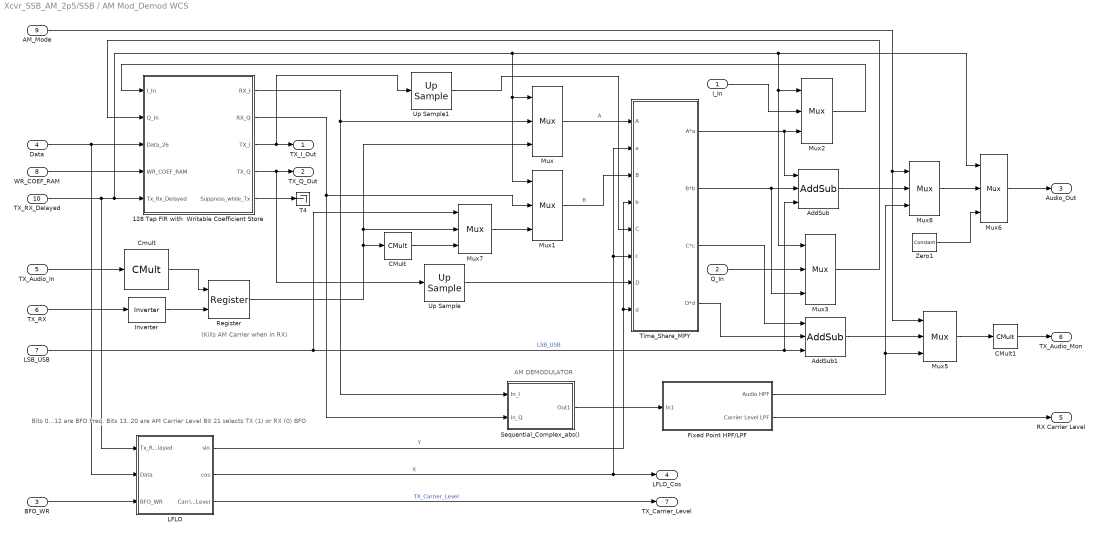
== system Xcvr_SSB_AM_2p5/SSB / AM Mod_Demod WCS ==
  note: Bits 0...12  are BFO Freq.
      | Bits 13..20 are AM Carrier Level
      | Bit 21 selects TX (1) or RX (0) BFO
  note: AM DEMODULATOR
  note: (Kills AM Carrier when in RX)
  I_In : Inport
  Q_In : Inport  Port=2
  BFO_WR : Inport  Port=3
  Data : Inport  Port=4
  TX_Audio_In : Inport  Port=5
  TX_RX : Inport  Port=6
  LSB_USB : Inport  Port=7
  WR_COEF_RAM : Inport  Port=8
  AM_Mode : Inport  Port=9
  TX_RX_Delayed : Inport  Port=10
  128 Tap FIR with  Writable Coefficient Store : Subsystem
  AddSub : xbsIndex_r4/AddSub  mode=Addition or Subtraction  use_carryin=off  use_carryout=off  en=off  latency=0  precision=User Defined  arith_type="Signed  (2's comp)"  n_bits=18  bin_pt=17  quantization="Round  (unbiased: +/- Inf)"  overflow=Wrap  dbl_ovrd=off  use_behavioral_HDL=off  hw_selection=Fabric  pipelined=off  use_rpm=on  block_type=addsub
      settings: block_version=9.2.00
  AddSub1 : xbsIndex_r4/AddSub  mode=Addition or Subtraction  use_carryin=off  use_carryout=off  en=off  latency=1  precision=User Defined  arith_type="Signed  (2's comp)"  n_bits=16  bin_pt=15  quantization="Round  (unbiased: +/- Inf)"  overflow=Wrap  dbl_ovrd=off  use_behavioral_HDL=off  hw_selection=Fabric  pipelined=off  use_rpm=on  block_type=addsub
      settings: block_version=9.2.00
  CMult : xbsIndex_r4/CMult  const=-1  gui_display_data_type=Fixed-point  const_n_bits=1  const_bin_pt=0  float_type=Single  exp_bits=8  fraction_bits=24  en=off  latency=0  precision=User Defined  arith_type="Signed  (2's comp)"  n_bits=16  bin_pt=15  quantization=Truncate  overflow=Wrap  dbl_ovrd=off  use_behavioral_HDL=off  mem_type=Distributed RAM  pipeline=off  use_rpm=off  placement_style=Rectangular Shape  block_type=cmult
      settings: block_version=9.2.00
  CMult1 : xbsIndex_r4/CMult  const=2  gui_display_data_type=Fixed-point  const_n_bits=3  const_bin_pt=0  float_type=Single  exp_bits=8  fraction_bits=24  en=off  latency=0  precision=User Defined  arith_type="Signed  (2's comp)"  n_bits=16  bin_pt=15  quantization=Truncate  overflow=Wrap  dbl_ovrd=off  use_behavioral_HDL=off  mem_type=Distributed RAM  pipeline=off  use_rpm=off  placement_style=Rectangular Shape  block_type=cmult
      settings: block_version=9.2.00
  Cmult : xbsIndex_r4/CMult  const=.5  gui_display_data_type=Fixed-point  const_n_bits=2  const_bin_pt=2  float_type=Single  exp_bits=8  fraction_bits=24  en=off  latency=0  precision=User Defined  arith_type="Signed  (2's comp)"  n_bits=16  bin_pt=15  quantization=Truncate  overflow=Wrap  dbl_ovrd=off  use_behavioral_HDL=off  mem_type=Distributed RAM  pipeline=off  block_type=cmult
      settings: block_version=12.1
  Fixed Point HPF/LPF : Subsystem  MinMaxOverflowLogging=MinMaxAndOverflow
  Inverter : xbsIndex_r4/Inverter  en=off  latency=0  dbl_ovrd=off  block_type=inv
      settings: block_version=12.1
  LFLO : Subsystem
  Mux{,1..3} (4 alike) : xbsIndex_r4/Mux  inputs=2  en=off  latency=0  precision=Full  arith_type=Unsigned  n_bits=16  bin_pt=14  quantization=Truncate  overflow=Wrap  dbl_ovrd=off  block_type=mux
      settings: block_version=9.2.00
  Mux5 : xbsIndex_r4/Mux  inputs=2  en=off  latency=0  precision=User Defined  arith_type="Signed  (2's comp)"  n_bits=16  bin_pt=15  quantization=Truncate  overflow=Wrap  dbl_ovrd=off  block_type=mux
      settings: block_version=9.2.00
  Mux6 : xbsIndex_r4/Mux  inputs=2  en=off  latency=0  precision=User Defined  arith_type="Signed  (2's comp)"  n_bits=18  bin_pt=17  quantization=Truncate  overflow=Wrap  dbl_ovrd=off  block_type=mux
      settings: block_version=9.2.00
  Mux7 : xbsIndex_r4/Mux  inputs=2  en=off  latency=0  precision=User Defined  arith_type="Signed  (2's comp)"  n_bits=16  bin_pt=15  quantization=Truncate  overflow=Wrap  dbl_ovrd=off  block_type=mux
      settings: block_version=9.2.00
  Mux8 : xbsIndex_r4/Mux  inputs=2  en=off  latency=0  precision=User Defined  arith_type="Signed  (2's comp)"  n_bits=18  bin_pt=17  quantization=Truncate  overflow=Wrap  dbl_ovrd=off  block_type=mux
      settings: block_version=9.2.00
  Register : xbsIndex_r4/Register  init=0  rst=on  en=off  dbl_ovrd=off  block_type=register
      settings: block_version=12.1
  Sequential_Complex_abs() : Subsystem
  T4 : Terminator
  Time_Share_MPY : Subsystem
  Up Sample : xbsIndex_r4/Up Sample  sample_ratio=64  copy_samples=off  en=off  latency=0  dbl_ovrd=off  block_type=usamp
  Up Sample1 : xbsIndex_r4/Up Sample  sample_ratio=64  copy_samples=off  en=off  latency=0  dbl_ovrd=off  block_type=usamp
  Zero1 : xbsIndex_r4/Constant  const=0  gui_display_data_type=Fixed-point  arith_type=Signed (2's comp)  n_bits=18  bin_pt=17  preci_type=Single  exp_width=8  frac_width=24  explicit_period=on  period=Daudio/Fs  equ=P=C  opselect=C  inp2=PCIN>>17  opr=+  inp1=P  carry=CIN  dbl_ovrd=off  block_type=constant
      settings: block_version=9.2.00
  TX_I_Out : Outport
  TX_Q_Out : Outport  Port=2
  Audio_Out : Outport  Port=3
  LFLO_Cos : Outport  Port=4
  RX Carrier Level : Outport  Port=5
  TX_Audio_Mon : Outport  Port=6
  TX_Carrier_Level : Outport  Port=7
  wires:
  LFLO/2(cos) -> LFLO_Cos/1, Time_Share_MPY/2(a), Time_Share_MPY/6(c)  "X"
  LFLO/1(sin) -> Time_Share_MPY/4(b), Time_Share_MPY/8(d)  "Y"
  LSB_USB/1 -> Mux7/1, AddSub/3, AddSub1/3  "LSB_USB"
  Mux/1 -> Time_Share_MPY/1(A)  "A"
  Mux1/1 -> Time_Share_MPY/3(B)  "B"
  128 Tap FIR with  Writable Coefficient Store/1(RX_I) -> Mux/2, Sequential_Complex_abs()/1(In_I)
  128 Tap FIR with  Writable Coefficient Store/2(RX_Q) -> Mux1/2, Sequential_Complex_abs()/2(In_Q)
  I_In/1 -> Mux2/2
  Mux2/1 -> 128 Tap FIR with  Writable Coefficient Store/1(I_In)
  Q_In/1 -> Mux3/2
  Mux3/1 -> 128 Tap FIR with  Writable Coefficient Store/2(Q_In)
  Mux7/1 -> Mux1/3
  CMult/1 -> Mux7/3
  Data/1 -> LFLO/2(Data), 128 Tap FIR with  Writable Coefficient Store/3(Data_26)
  BFO_WR/1 -> LFLO/3(BFO_WR)
  Mux6/1 -> Audio_Out/1
  Zero1/1 -> Mux6/3
  TX_RX_Delayed/1 -> Mux6/1, Mux3/1, Mux2/1, Mux1/1, Mux/1, 128 Tap FIR with  Writable Coefficient Store/5(Tx_Rx_Delayed), LFLO/1(Tx_Rx_Delayed)
  WR_COEF_RAM/1 -> 128 Tap FIR with  Writable Coefficient Store/4(WR_COEF_RAM)
  Fixed Point HPF/LPF/1(Audio HPF) -> Mux8/3, Mux5/3
  Fixed Point HPF/LPF/2(Carrier Level LPF) -> RX Carrier Level/1
  AM_Mode/1 -> Mux5/1, Mux8/1
  AddSub/1 -> Mux8/2
  Mux8/1 -> Mux6/2
  LFLO/3(Carrier_Level) -> TX_Carrier_Level/1  "TX_Carrier_Level"
  128 Tap FIR with  Writable Coefficient Store/3(TX_I) -> Up Sample1/1, TX_I_Out/1
  128 Tap FIR with  Writable Coefficient Store/4(TX_Q) -> Up Sample/1, TX_Q_Out/1
  Sequential_Complex_abs()/1(Out1) -> Fixed Point HPF/LPF/1(In1)
  Inverter/1 -> Register/2
  TX_RX/1 -> Inverter/1
  Cmult/1 -> Register/1
  Register/1 -> CMult/1, Mux/3, Mux7/2
  128 Tap FIR with  Writable Coefficient Store/5(Suppress_while_Tx) -> T4/1
  TX_Audio_In/1 -> Cmult/1
  Time_Share_MPY/1(A*a) -> AddSub/1, Mux2/3
  Time_Share_MPY/2(B*b) -> AddSub/2, Mux3/3
  Time_Share_MPY/3(C*c) -> AddSub1/1
  Time_Share_MPY/4(D*d) -> AddSub1/2
  AddSub1/1 -> Mux5/2
  CMult1/1 -> TX_Audio_Mon/1
  Mux5/1 -> CMult1/1
  Up Sample/1 -> Time_Share_MPY/7(D)
  Up Sample1/1 -> Time_Share_MPY/5(C)
